simulink model "ObiektARMAX"  (Simulink 9.1)
settings: Solver=FixedStepDiscrete  StartTime=0.0  StopTime=tend  FixedStep=Tp  RelTol=1e-3  EnableMultiTasking=on
values from neighbouring files (symbols this model uses):
  c10 = 0    [ZAD1_1_skrypt.m]    (also in ZAD1_2_skrypt.m = 0.7; ZAD2_1_skrypt.m = 0.7)
  Td = 1500    [ZAD1_1_skrypt.m]    (also in ZAD1_2_skrypt.m; ZAD2_1_skrypt.m = 300)
  Tp = 0.1    [ZAD1_1_skrypt.m]    (also in ZAD1_2_skrypt.m; ZAD2_1_skrypt.m)
libraries: simulink x1
settings Model: Creator=szymon  LastModifiedBy=szymon
settings DataIOCC: LimitDataPoints=on  SignalLoggingSaveFormat=ModelDataLogs
settings OptimizationCC: InitFltsAndDblsToZero=on
settings DebuggingCC: SaveWithParameterizedLinksMsg=none  SignalResolutionControl=TryResolveAllWithWarning  SolverPrmCheckMsg=warning  MultiTaskDSMMsg=warning  MultiTaskCondExecSysMsg=none  FcnCallInpInsideContextMsg=warning
settings GRTTargetCC: TargetFcnLib=ansi_tfl_tmw.mat

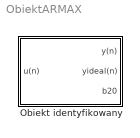
== system ObiektARMAX ==
  Obiekt identyfikowany : Subsystem

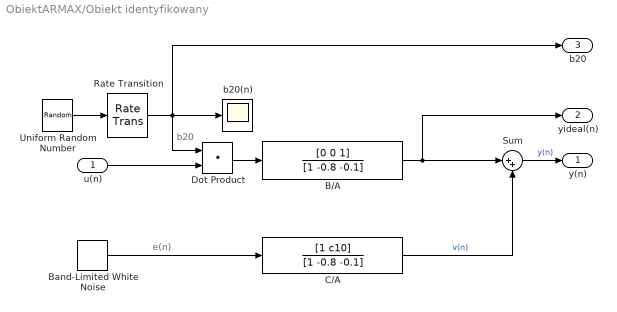
== system ObiektARMAX/Obiekt identyfikowany ==
  note: b20
  note: e(n)
  u(n) : Inport
  B/A : DiscreteFilter  Numerator=[0 0 1]  Denominator=[1 -0.8 -0.1]  SampleTime=Tp
  Band-Limited White Noise : simulink/Sources/Band-Limited White Noise  Cov=[0.001]  Ts=Tp  seed=[23341]
  C/A : DiscreteFilter  Numerator=[1 c10]  Denominator=[1 -0.8 -0.1]  SampleTime=Tp
  Dot Product : DotProduct  InputSameDT=on  OutDataTypeStr=Inherit: Inherit via internal rule
  Rate Transition : RateTransition  InitialCondition=0.5  OutPortSampleTime=Tp
  Sum : Sum  Inputs=|++  SaturateOnIntegerOverflow=on
  Uniform Random Number : UniformRandomNumber  Minimum=0  Maximum=0.5  SampleTime=Td
  b20(n) : Scope
  y(n) : Outport
  yideal(n) : Outport  Port=2
  b20 : Outport  Port=3
  wires:
  C/A/1 -> Sum/2  "v(n)"
  Sum/1 -> y(n)/1  "y(n)"
  Band-Limited White Noise/1 -> C/A/1
  B/A/1 -> yideal(n)/1, Sum/1
  u(n)/1 -> Dot Product/2
  Dot Product/1 -> B/A/1
  Uniform Random Number/1 -> Rate Transition/1
  Rate Transition/1 -> Dot Product/1, b20(n)/1, b20/1
